simulink model "dF_test"  (R2016b)
settings: Solver=VariableStepAuto  StartTime=0.0  StopTime=2^16/Fadc  RelTol=1e-3  EnableMultiTasking=on
PreLoadFcn:
  | setup
values from neighbouring files (symbols this model uses):
  Fadc = 614.4e6    (= 614400000)    [setup.m]
libraries: xbsIndex_r4 x12, dspsigops x2, simulink x1, CryoDetLibCMB x1
settings Model: Creator=Mitch  LastModifiedBy=mdewart
settings OptimizationCC: LifeSpan=inf
settings DebuggingCC: SFUnexpectedBacktrackingDiag=warning  SFNoUnconditionalDefaultTransitionDiag=warning  SFExecutionAtInitializationDiag=none
settings GRTTargetCC: TargetLangStandard=C89/C90 (ANSI)  GeneratePreprocessorConditionals=Disable all
settings ConfigComp: CovMetricSettings=dw  CovHtmlReporting=on  CovSaveCumulativeToWorkspaceVar=on  CovSaveSingleToWorkspaceVar=on  CovExternalEMLEnable=off

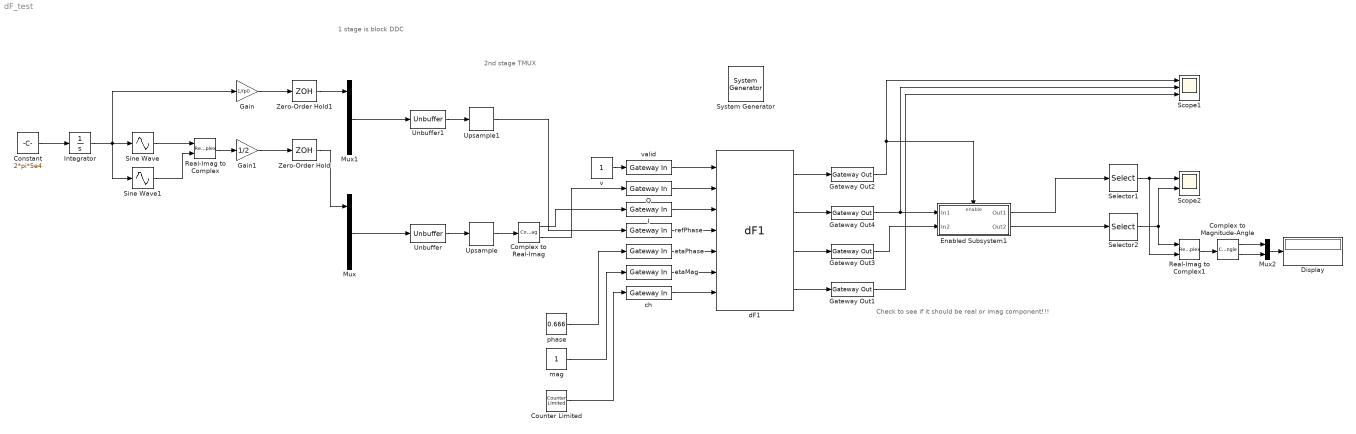
== system dF_test ==
  note: 2nd stage TMUX
  note: 1 stage is block DDC
  note: Check to see if it should be real or imag component!!!
  " System Generator" : xbsIndex_r4/ System Generator  Tag=genX  xilinxfamily=kintexu  part=xcku040  speed=-2-e  package=ffva1156  synthesis_tool=Vivado  clock_wrapper=Clock Enables  directory=./netlist  proj_type=Vivado  Synth_file=Vivado Synthesis Defaults  Impl_file=Vivado Implementation Defaults  testbench=off  simulink_period=2/Fadc  sysclk_period=2e9/Fadc  dcm_input_clock_period=10  incr_netlist=off  trim_vbits=Everywhere in SubSystem  dbl_ovrd=According to Block Masks  core_generation=According to Block Masks  run_coregen=off  deprecated_control=off  eval_field=0  block_type=sysgen
  Complex to Magnitude-Angle : ComplexToMagnitudeAngle
  Complex to Real-Imag : ComplexToRealImag
  Constant : Constant  Value=2*pi*5e4
  Counter Limited : simulink/Sources/Counter Limited  uplimit=127  tsamp=2/Fadc
  Display : Display
  Enabled Subsystem1 : Subsystem  TreatAsAtomicUnit=on
  Gain : Gain  Gain=1/(pi)
  Gain1 : Gain  Gain=1/2
  Gateway Out{1..4} (4 alike) : xbsIndex_r4/Gateway Out  inherit_from_input=off  hdl_port=on  rows=1  columns=1  UseAsDAC=off  DACChannel='1'  interface=None  automatic_assignment=on  address_offset=hex2dec('00')  intf_name=''  intf_description=''  timing_constraint=None  locs_specified=off  LOCs={}  io_standard={}  block_type=gatewayout
  I : xbsIndex_r4/Gateway In  gui_display_data_type=Fixed-point  arith_type="Signed  (2's comp)"  n_bits=18  bin_pt=16  preci_type=Single  exp_width=8  frac_width=24  rows=1  columns=1  quantization="Round  (unbiased: +/- Inf)"  overflow=Saturate  period=2/Fadc  UseAsADC=off  ADCChannel='1'  interface=None  automatic_assignment=on  address_offset=hex2dec('00')  intf_name=''  intf_description=''  default_value=0  timing_constraint=None  locs_specified=off  LOCs={}  io_standard={}  inherit_from_input=off  hdl_port=on  dbl_ovrd=off  block_type=gatewayin
  Integrator : Integrator
  Mux : Mux  Inputs=16
  Mux1 : Mux  Inputs=16
  Mux2 : Mux  Inputs=2
  Q : xbsIndex_r4/Gateway In  gui_display_data_type=Fixed-point  arith_type="Signed  (2's comp)"  n_bits=18  bin_pt=16  preci_type=Single  exp_width=8  frac_width=24  rows=1  columns=1  quantization="Round  (unbiased: +/- Inf)"  overflow=Saturate  period=2/Fadc  UseAsADC=off  ADCChannel='1'  interface=None  automatic_assignment=on  address_offset=hex2dec('00')  intf_name=''  intf_description=''  default_value=0  timing_constraint=None  locs_specified=off  LOCs={}  io_standard={}  inherit_from_input=off  hdl_port=on  dbl_ovrd=off  block_type=gatewayin
  Real-Imag to Complex : RealImagToComplex
  Real-Imag to Complex1 : RealImagToComplex
  Scope1 : Scope  NumInputPorts=3
  Scope2 : Scope  NumInputPorts=2
  Selector1 : Selector  InputPortWidth=128  IndexOptions=Index vector (dialog)  Indices=[1]  OutputSizes=1
  Selector2 : Selector  InputPortWidth=128  IndexOptions=Index vector (dialog)  Indices=[1]  OutputSizes=1
  Sine Wave : Sin  TimeSource=Use external signal  Phase=-pi/3  SampleTime=256/Fadc
  Sine Wave1 : Sin  TimeSource=Use external signal  Phase=-pi/2-pi/3  SampleTime=256/Fadc
  Unbuffer : Unbuffer  SampleBasedProcessing=Same as frame based
  Unbuffer1 : Unbuffer  SampleBasedProcessing=Same as frame based
  Upsample : dspsigops/Upsample  N=8  phase=0  RateOptions=Allow multirate processing  ic=0  mode=Unused parameter value
  Upsample1 : dspsigops/Upsample  N=8  phase=0  RateOptions=Allow multirate processing  ic=0  mode=Unused parameter value
  Zero-Order Hold : ZeroOrderHold  SampleTime=256/Fadc
  Zero-Order Hold1 : ZeroOrderHold  SampleTime=256/Fadc
  ch : xbsIndex_r4/Gateway In  gui_display_data_type=Fixed-point  arith_type=Unsigned  n_bits=7  bin_pt=0  preci_type=Single  exp_width=8  frac_width=24  rows=1  columns=1  quantization="Round  (unbiased: +/- Inf)"  overflow=Saturate  period=2/Fadc  UseAsADC=off  ADCChannel='1'  interface=None  automatic_assignment=on  address_offset=hex2dec('00')  intf_name=''  intf_description=''  default_value=0  timing_constraint=None  locs_specified=off  LOCs={}  io_standard={}  inherit_from_input=off  hdl_port=on  dbl_ovrd=off  block_type=gatewayin
  dF1 : CryoDetLibCMB/dF1
  etaMag : xbsIndex_r4/Gateway In  gui_display_data_type=Fixed-point  arith_type=Unsigned  n_bits=16  bin_pt=10  preci_type=Single  exp_width=8  frac_width=24  rows=1  columns=1  quantization="Round  (unbiased: +/- Inf)"  overflow=Saturate  period=2/Fadc  UseAsADC=off  ADCChannel='1'  interface=None  automatic_assignment=on  address_offset=hex2dec('00')  intf_name=''  intf_description=''  default_value=0  timing_constraint=None  locs_specified=off  LOCs={}  io_standard={}  inherit_from_input=off  hdl_port=on  dbl_ovrd=off  block_type=gatewayin
  etaPhase : xbsIndex_r4/Gateway In  gui_display_data_type=Fixed-point  arith_type="Signed  (2's comp)"  n_bits=16  bin_pt=15  preci_type=Single  exp_width=8  frac_width=24  rows=1  columns=1  quantization="Round  (unbiased: +/- Inf)"  overflow=Saturate  period=2/Fadc  UseAsADC=off  ADCChannel='1'  interface=None  automatic_assignment=on  address_offset=hex2dec('00')  intf_name=''  intf_description=''  default_value=0  timing_constraint=None  locs_specified=off  LOCs={}  io_standard={}  inherit_from_input=off  hdl_port=on  dbl_ovrd=off  block_type=gatewayin
  mag : Constant  SampleTime=2/Fadc
  phase : Constant  Value=0.666  SampleTime=2/Fadc
  refPhase : xbsIndex_r4/Gateway In  gui_display_data_type=Fixed-point  arith_type="Signed  (2's comp)"  n_bits=16  bin_pt=15  preci_type=Single  exp_width=8  frac_width=24  rows=1  columns=1  quantization="Round  (unbiased: +/- Inf)"  overflow=Wrap  period=2/Fadc  UseAsADC=off  ADCChannel='1'  interface=None  automatic_assignment=on  address_offset=hex2dec('00')  intf_name=''  intf_description=''  default_value=0  timing_constraint=None  locs_specified=off  LOCs={}  io_standard={}  inherit_from_input=off  hdl_port=on  dbl_ovrd=off  block_type=gatewayin
  v : Constant  SampleTime=2/Fadc
  valid : xbsIndex_r4/Gateway In  gui_display_data_type=Boolean  arith_type=Boolean  n_bits=18  bin_pt=15  preci_type=Single  exp_width=8  frac_width=24  rows=1  columns=1  quantization="Round  (unbiased: +/- Inf)"  overflow=Saturate  period=2/Fadc  UseAsADC=off  ADCChannel='1'  interface=None  automatic_assignment=on  address_offset=hex2dec('00')  intf_name=''  intf_description=''  default_value=0  timing_constraint=None  locs_specified=off  LOCs={}  io_standard={}  inherit_from_input=off  hdl_port=on  dbl_ovrd=off  block_type=gatewayin
  wires:
  Mux/1 -> Unbuffer/1
  Unbuffer/1 -> Upsample/1
  Counter Limited/1 -> ch/1
  Sine Wave/1 -> Real-Imag to Complex/1
  Real-Imag to Complex/1 -> Gain1/1
  Sine Wave1/1 -> Real-Imag to Complex/2
  dF1/3 -> Gateway Out3/1
  dF1/2 -> Gateway Out4/1
  dF1/1 -> Gateway Out2/1
  Gateway Out4/1 -> Enabled Subsystem1/1(In1), Scope1/2
  Enabled Subsystem1/1(Out1) -> Selector1/1
  Enabled Subsystem1/2(Out2) -> Selector2/1
  Selector1/1 -> Real-Imag to Complex1/2, Scope2/1
  Selector2/1 -> Real-Imag to Complex1/1, Scope2/2
  phase/1 -> etaPhase/1
  Zero-Order Hold/1 -> Mux/1
  Constant/1 -> Integrator/1
  Complex to Real-Imag/1 -> I/1
  Complex to Real-Imag/2 -> Q/1
  Mux1/1 -> Unbuffer1/1
  Unbuffer1/1 -> Upsample1/1
  Zero-Order Hold1/1 -> Mux1/1
  Integrator/1 -> Gain/1, Sine Wave1/1, Sine Wave/1
  Upsample/1 -> Complex to Real-Imag/1
  Gain/1 -> Zero-Order Hold1/1
  Upsample1/1 -> refPhase/1
  Gain1/1 -> Zero-Order Hold/1
  Real-Imag to Complex1/1 -> Complex to Magnitude-Angle/1
  Complex to Magnitude-Angle/1 -> Mux2/1
  Complex to Magnitude-Angle/2 -> Mux2/2
  Mux2/1 -> Display/1
  dF1/4 -> Gateway Out1/1
  Gateway Out1/1 -> Scope1/3
  I/1 -> dF1/3
  Q/1 -> dF1/2
  valid/1 -> dF1/1
  refPhase/1 -> dF1/4
  etaMag/1 -> dF1/6
  etaPhase/1 -> dF1/5
  ch/1 -> dF1/7
  v/1 -> valid/1
  mag/1 -> etaMag/1
  Gateway Out2/1 -> Enabled Subsystem1/Enable, Scope1/1
  Gateway Out3/1 -> Enabled Subsystem1/2(In2)

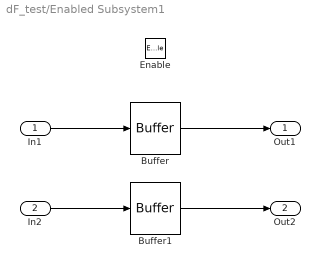
== system dF_test/Enabled Subsystem1 ==
  In1 : Inport
  In2 : Inport  Port=2
  Enable : EnablePort
  Buffer : Buffer  N=128  TreatMby1Signals=One channel  OutputFrames=off
  Buffer1 : Buffer  N=128  TreatMby1Signals=One channel  OutputFrames=off
  Out1 : Outport
  Out2 : Outport  Port=2
  wires:
  Buffer/1 -> Out1/1
  In1/1 -> Buffer/1
  Buffer1/1 -> Out2/1
  In2/1 -> Buffer1/1
